simulink model "IMU_test"  (Simulink 7.6)
settings: Solver=FixedStepDiscrete  StartTime=0.0  StopTime=Inf  RelTol=1e-3
libraries: rpi_blkst x1
settings Model: Creator=jacques  LastModifiedBy=jacques  SimulationMode=external
settings OptimizationCC: OptimizeModelRefInitCode=on  LifeSpan=1
settings HardwareCC: ProdIntDivRoundTo=Zero  ProdEndianess=LittleEndian  ProdHWDeviceType=Intel->x86/Pentium
settings RTWCC: SystemTargetFile=ert_rpi.tlc  TemplateMakefile=ert_rpi.tmf  PostCodeGenCommand=postGenFunc(buildInfo)  Description=RTW Embedded Coder RPI target  ProcessScript=ert_rpi_make_rtw_hook
settings CodeAppCC: IgnoreCustomStorageClasses=off
settings STFCustomTargetCC: ModelReferenceCompliant=off  CombineOutputUpdateFcns=on  ERTCustomFileBanners=on  SupportNonInlinedSFcns=off  SystemTargetFile=ert_rpi.tlc
settings ERTTargetCC: MultiwordLength=2048  ModelReferenceCompliant=off  ParMdlRefBuildCompliant=off  CompOptLevelCompliant=off  ERTFirstTimeCompliant=off  SupportContinuousTime=on  ModelStepFunctionPrototypeControlCompliant=off  CPPClassGenCompliant=off  ExtMode=on  ExtModeMexArgs='192.168.2.1'  InlinedParameterPlacement=NonHierarchical  ERTCustomFileTemplate=ert_rpi_file_process.tlc  ConvertIfToSwitch=off

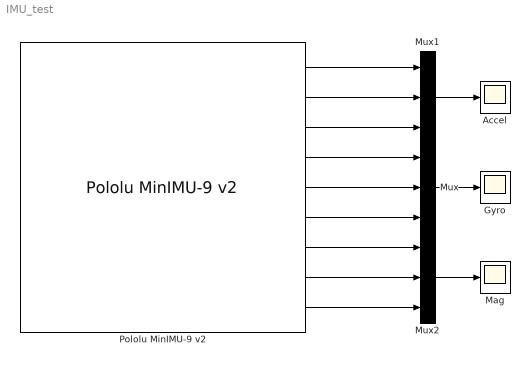
== system IMU_test ==
  Accel : Scope
      settings: YMin=-1.5  YMax=0.7
  Gyro : Scope
      settings: YMin=-50  YMax=80
  Mag : Scope
      settings: YMin=-0.15  YMax=0.5  SaveName=ScopeData2
  Mux : Mux  Inputs=3
  Mux1 : Mux  Inputs=3
  Mux2 : Mux  Inputs=3
  Pololu MinIMU-9 v2 : rpi_blkst/Pololu MinIMU-9 v2  SystemSampleTime=-1  rpi_mask_Ts=0.01
  wires:
  Pololu MinIMU-9 v2/9 -> Mux2/3
  Pololu MinIMU-9 v2/8 -> Mux2/2
  Pololu MinIMU-9 v2/7 -> Mux2/1
  Pololu MinIMU-9 v2/1 -> Mux1/1
  Pololu MinIMU-9 v2/2 -> Mux1/2
  Pololu MinIMU-9 v2/3 -> Mux1/3
  Pololu MinIMU-9 v2/4 -> Mux/1
  Pololu MinIMU-9 v2/5 -> Mux/2
  Pololu MinIMU-9 v2/6 -> Mux/3
  Mux/1 -> Gyro/1
  Mux1/1 -> Accel/1
  Mux2/1 -> Mag/1
